simulink model "Recursive_Moving_Average"  (R2017a)
settings: Solver=VariableStepAuto  StartTime=0.0  StopTime=0.1  RelTol=1e-3
StopFcn:
  | dlmwrite("TestData.csv", [round(filter_input.time*1000000), round(filter_input.data), round(filter_output.data)], 'precision', '%i')
settings Model: Creator=Max  LastModifiedBy=Max

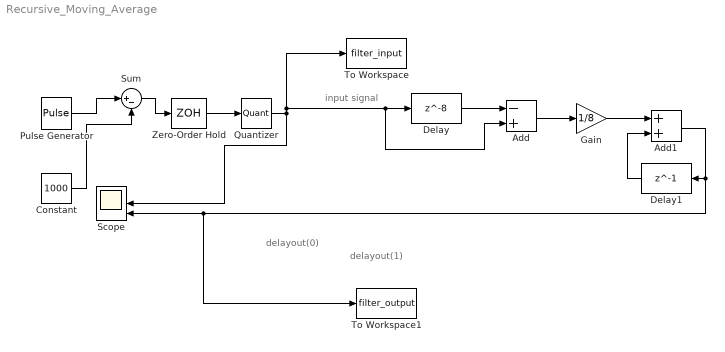
== system Recursive_Moving_Average ==
  note: delayout(1)
  note: input signal
  note: delayout(0)
  Add : Sum  Inputs=-+
  Add1 : Sum
  Constant : Constant  Value=1000
  Delay : Delay  DelayLength=8  SampleTime=1e-3
  Delay1 : Delay  DelayLength=1  SampleTime=1e-3
  Gain : Gain  Gain=1/8
  Pulse Generator : DiscretePulseGenerator  PulseType=Time based  Amplitude=3000  Period=0.008  PulseWidth=50
  Quantizer : Quantizer  QuantizationInterval=0.000244140625
  Scope : Scope  NumInputPorts=3
  Sum : Sum  Inputs=|+-
  To Workspace : ToWorkspace  VariableName=filter_input  SaveFormat=Timeseries  SampleTime=-1
  To Workspace1 : ToWorkspace  VariableName=filter_output  SaveFormat=Timeseries  SampleTime=-1
  Zero-Order Hold : ZeroOrderHold  SampleTime=1e-3
  wires:
  Quantizer/1 -> Add/2, Delay/1, To Workspace/1, Scope/2
  Zero-Order Hold/1 -> Quantizer/1
  Add1/1 -> Delay1/1, To Workspace1/1, Scope/3
  Delay/1 -> Add/1
  Add/1 -> Gain/1
  Gain/1 -> Add1/1
  Delay1/1 -> Add1/2
  Pulse Generator/1 -> Sum/1
  Sum/1 -> Zero-Order Hold/1
  Constant/1 -> Sum/2
